simulink model "guiji_6d1"  (R2018b)
settings: Solver=ode45  StartTime=0.0  StopTime=2  RelTol=1e-3  EnableMultiTasking=on
settings Model: Creator=YuXiaozhi  LastModifiedBy=Lenovo
settings DataIOCC: LimitDataPoints=on  SaveFormat=Array
settings OptimizationCC: LifeSpan=inf
settings DebuggingCC: SolverPrmCheckMsg=warning  SFUnexpectedBacktrackingDiag=warning  SFNoUnconditionalDefaultTransitionDiag=warning  SFExecutionAtInitializationDiag=none
settings HardwareCC: ProdBitPerPointer=32  ProdBitPerSizeT=32  ProdBitPerPtrDiffT=32  ProdLargestAtomicFloat=None  ProdIntDivRoundTo=Undefined  ProdEndianess=Unspecified  ProdWordSize=32  ProdHWDeviceType=32-bit Generic
settings ModelReferenceCC: PropagateSignalLabelsOutOfModel=off
settings SFSimCC: SimUseLocalCustomCode=off
settings RTWCC: RTWUseLocalCustomCode=off
settings CodeAppCC: StateflowObjectComments=on
settings GRTTargetCC: TargetLangStandard=C89/C90 (ANSI)  GeneratePreprocessorConditionals=Disable all
settings ConfigComp: CovMetricSettings=dw  CovHtmlReporting=on  CovSaveCumulativeToWorkspaceVar=on  CovSaveSingleToWorkspaceVar=on  CovExternalEMLEnable=off  CovSFcnEnable=off

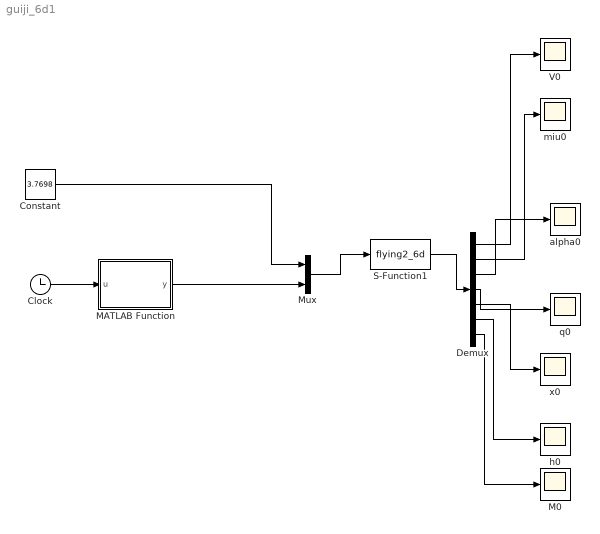
== system guiji_6d1 ==
  Clock : Clock
  Constant : Constant  Value=3.7698
  Demux : Demux  Outputs=7
  M0 : Scope
  MATLAB Function : MATLAB Function  TreatAsAtomicUnit=on
  Mux : Mux  Inputs=2
  S-Function1 : S-Function  FunctionName=flying2_6d  SFunctionDeploymentMode=off  EnableBusSupport=off
  V0 : Scope
  alpha0 : Scope
  h0 : Scope
  miu0 : Scope
  q0 : Scope
  x0 : Scope
  wires:
  Mux/1 -> S-Function1/1
  Clock/1 -> MATLAB Function/1(u)
  MATLAB Function/1(y) -> Mux/2
  Constant/1 -> Mux/1
  S-Function1/1 -> Demux/1
  Demux/1 -> V0/1
  Demux/2 -> miu0/1
  Demux/3 -> alpha0/1
  Demux/4 -> q0/1
  Demux/5 -> x0/1
  Demux/6 -> h0/1
  Demux/7 -> M0/1

== matlab function guiji_6d1/MATLAB Function ==
  data: u input; y output
function y = fcn(u)
if u<0.3
    y=-(11+(u)/0.3*22)/180*pi;
else if u>=0.3&&u<0.5
        y=-(33+(u-0.3)/0.2*15)/180*pi;
else if u>=0.5&&u<0.7
        y=-(33+15-(u-0.5)/0.2*30)/180*pi;   
    else
        y=-(18)/180*pi;
    end
    end
end
